simulink model "Lagged_FlowValve"  (R2021b)
settings: Solver=VariableStepAuto  StartTime=0.0  StopTime=10.0  RelTol=1e-3
settings Model: Creator=Edwar  LastModifiedBy=Edwar

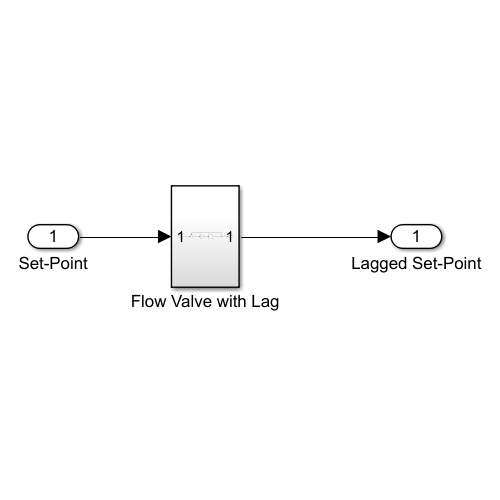
[thumbnail: Simulink's stored preview of the top-level diagram]
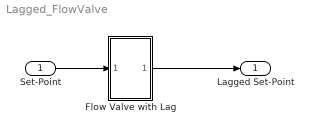
== system Lagged_FlowValve ==
  Set-Point : Inport
  Flow Valve with Lag : Subsystem
  Lagged Set-Point : Outport
  wires:
  Set-Point/1 -> Flow Valve with Lag/1(In1)
  Flow Valve with Lag/1(Out1) -> Lagged Set-Point/1

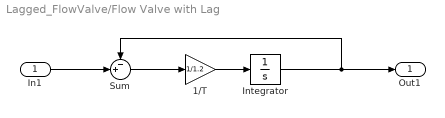
== system Lagged_FlowValve/Flow Valve with Lag ==
  In1 : Inport
  1/T : Gain  Gain=1/1.2
  Integrator : Integrator
  Sum : Sum  Inputs=-+|
  Out1 : Outport
  wires:
  Integrator/1 -> Out1/1, Sum/1
  Sum/1 -> 1/T/1
  1/T/1 -> Integrator/1
  In1/1 -> Sum/2
